simulink model "Gain_Multiplication"  (R2025a)
settings: Solver=VariableStepAuto  StartTime=0.0  StopTime=10.0  MaxStep=0.01  RelTol=1e-3
settings Model: Creator=Pablo  LastModifiedBy=Pablo

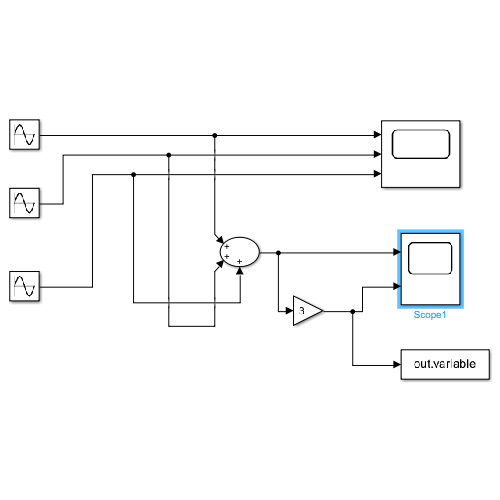
[thumbnail: Simulink's stored preview of the top-level diagram]
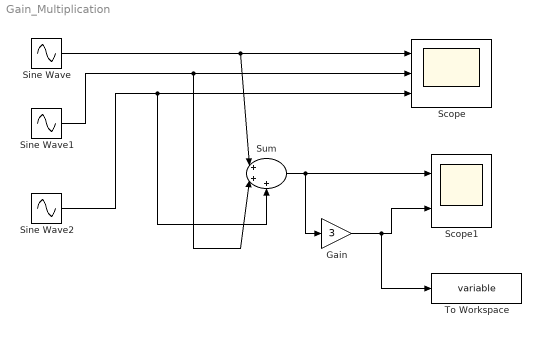
== system Gain_Multiplication ==
  Gain : Gain  Gain=3
  Scope : Scope  NumInputPorts=3
      settings: ActiveDisplayYMinimum=-1.2499967500526621  ActiveDisplayYMaximum=1.2499992865967788
  Scope1 : Scope  NumInputPorts=2
      settings: ActiveDisplayYMinimum=-4.8717440554302893  ActiveDisplayYMaximum=6.3691666183678119
  Sine Wave : Sin  SampleTime=0
  Sine Wave1 : Sin  Frequency=5  SampleTime=0
  Sine Wave2 : Sin  Frequency=10  SampleTime=0
  Sum : Sum  Inputs=|+++
  To Workspace : ToWorkspace  VariableName=variable  SaveFormat=Timeseries  SampleTime=-1
  wires:
  Sine Wave/1 -> Scope/1, Sum/1
  Sine Wave1/1 -> Scope/2, Sum/2
  Sine Wave2/1 -> Scope/3, Sum/3
  Sum/1 -> Gain/1, Scope1/1
  Gain/1 -> To Workspace/1, Scope1/2
